simulink model "basic_pid"  (R2020a)
settings: Solver=VariableStepAuto  StartTime=0.0  StopTime=10.0  RelTol=1e-3
libraries: simulink x1
settings Model: Creator=ripme  LastModifiedBy=ripme
settings SolverCC: ZeroCrossAlgorithm=Adaptive
settings DebuggingCC: IgnoredZcDiagnostic=none

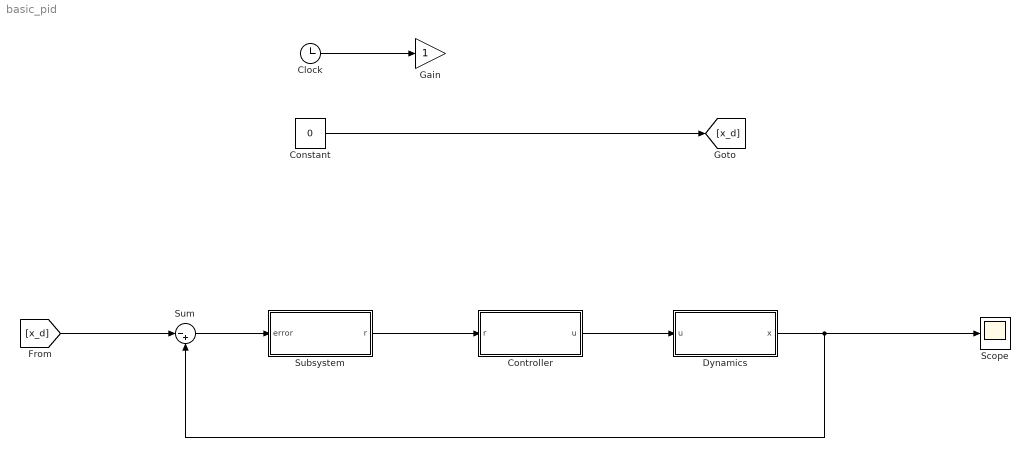
== system basic_pid ==
  Clock : Clock
  Constant : Constant  Value=0
  Controller : Subsystem
  Dynamics : Subsystem
  Gain : Gain
  Scope : Scope
  Subsystem : Subsystem
  Sum : Sum  Inputs=|-+
  wires:
  Controller/1(u) -> Dynamics/1(u)
  [x_d] -> Sum/1
  Dynamics/1(x) -> Scope/1, Sum/2
  Clock/1 -> Gain/1
  Subsystem/1(r) -> Controller/1(r)
  Sum/1 -> Subsystem/1(error)
  Constant/1 -> [x_d]

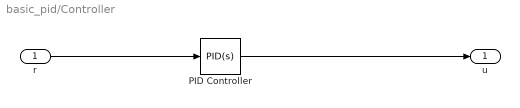
== system basic_pid/Controller ==
  r : Inport
  PID Controller : simulink/Continuous/PID Controller  Controller=PID  Form=Parallel  TimeDomain=Continuous-time  UseExternalTs=off  SampleTime=-1  IntegratorMethod=Forward Euler  FilterMethod=Forward Euler  ControllerParametersSource=internal  P=-4.49017102989629  I=-8.27054182231017  D=-0.547590052985724  UseFilter=on  N=322.390213985937  TunerSelectOption=Transfer Function Based (PID Tuner App)  InitialConditionSource=internal  InitialConditionForIntegrator=0  InitialConditionForFilter=0  DifferentiatorICPrevScaledInput=0  ExternalReset=none  TrackingMode=off  Kt=1  LimitOutput=off  UpperSaturationLimit=inf  LowerSaturationLimit=-inf  LinearizeAsGain=on  AntiWindupMode=none  Kb=1  POutMin=[]  POutMax=[]  IOutMin=[]  IOutMax=[]  DOutMin=[]  DOutMax=[]  NOutMin=[]  NOutMax=[]  SumOutMin=[]  SumOutMax=[]  SaturationOutMin=[]  SaturationOutMax=[]  PParamMin=[]  PParamMax=[]  IParamMin=[]  IParamMax=[]  DParamMin=[]  DParamMax=[]  NParamMin=[]  NParamMax=[]  KbParamMin=[]  KbParamMax=[]  KtParamMin=[]  KtParamMax=[]  KbOutMin=[]  KbOutMax=[]  KtOutMin=[]  KtOutMax=[]  IntegratorOutMin=[]  IntegratorOutMax=[]  FilterOutMin=[]  FilterOutMax=[]  SumI1OutMin=[]  SumI1OutMax=[]  SumI2OutMin=[]  SumI2OutMax=[]  SumI3OutMin=[]  SumI3OutMax=[]  SumI4OutMin=[]  SumI4OutMax=[]  SumDOutMin=[]  SumDOutMax=[]  DifferentiatorOutMin=[]  DifferentiatorOutMax=[]  FilterDiffOutCoefMin=[]  FilterDiffOutCoefMax=[]  ReciprocalOutMin=[]  ReciprocalOutMax=[]  SumDenOutMin=[]  SumDenOutMax=[]  SumNumOutMin=[]  SumNumOutMax=[]  DivideOutMin=[]  DivideOutMax=[]  UdiffTsProdOutMin=[]  UdiffTsProdOutMax=[]  NTsProdOutMin=[]  NTsProdOutMax=[]  UintegralTsProdOutMin=[]  UintegralTsProdOutMax=[]  UngainTsProdOutMin=[]  UngainTsProdOutMax=[]  IntegratorContinuousStateAttributes=''  IntegratorStateMustResolveToSignalObject=off  IntegratorRTWStateStorageClass=Auto  FilterContinuousStateAttributes=''  FilterStateMustResolveToSignalObject=off  FilterRTWStateStorageClass=Auto  ParallelPVariant=InternalParameters  IdealPVariant=Disabled  IVariant=InternalParameters  DVariant=InternalParameters  IntegratorVariant=Continuous  SatVariant=Disabled  AWVariant=Passthrough  PCopyVariant=Disabled  TRVariant=Disabled  FdbkBlocksVariant=Forward  IdealPFdbkVariant=Disabled  SatFdbkVariant=Disabled  DerivativeFilterVariant=ContFilter  NVariant=InternalParameters  NCopyVariant=Disabled  FilterICVariant=InternalICsFilter  IntegratorICVariant=InternalICs  ExternalResetVariant=Disabled  TRSumVariant=Passthrough  SumFdbkVariant=Disabled  SumVariant=Sum_PID  TsampFilterVariant=InternalTs  TsampNgainVariant=Passthrough  TsampIntegralVariant=Passthrough
  u : Outport
  wires:
  PID Controller/1 -> u/1
  r/1 -> PID Controller/1

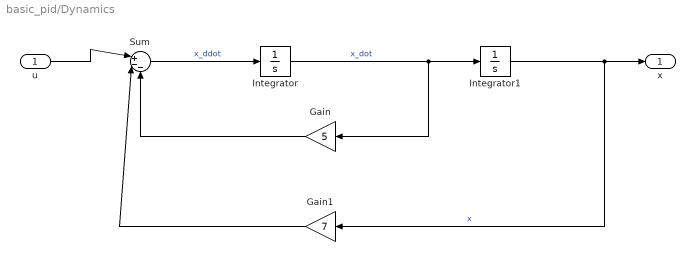
== system basic_pid/Dynamics ==
  u : Inport
  Gain : Gain  Gain=5
  Gain1 : Gain  Gain=7
  Integrator : Integrator  InitialCondition=5
  Integrator1 : Integrator  InitialCondition=5
  Sum : Sum  Inputs=|+--
  x : Outport
  wires:
  Sum/1 -> Integrator/1  "x_ddot"
  Integrator/1 -> Gain/1, Integrator1/1  "x_dot"
  Integrator1/1 -> Gain1/1, x/1  "x"
  u/1 -> Sum/1
  Gain/1 -> Sum/3
  Gain1/1 -> Sum/2

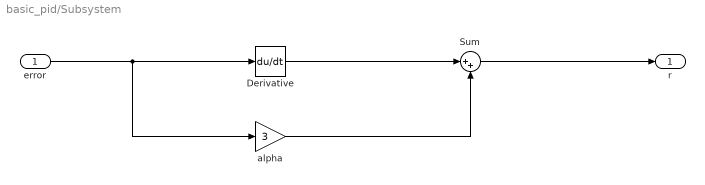
== system basic_pid/Subsystem ==
  error : Inport
  Derivative : Derivative
  Sum : Sum  Inputs=|++
  alpha : Gain  Gain=3
  r : Outport
  wires:
  alpha/1 -> Sum/2
  Sum/1 -> r/1
  Derivative/1 -> Sum/1
  error/1 -> alpha/1, Derivative/1
